simulink model "single_phase_csi"  (Simulink 6.1)
settings: Solver=ode23tb  StartTime=0.0  StopTime=0.03  MaxStep=1e-5  RelTol=1e-3  AbsTol=.01
libraries: powerlib x11
settings Model: LastModifiedBy=ThinkPad
settings DebuggingCC: SolverPrmCheckMsg=warning

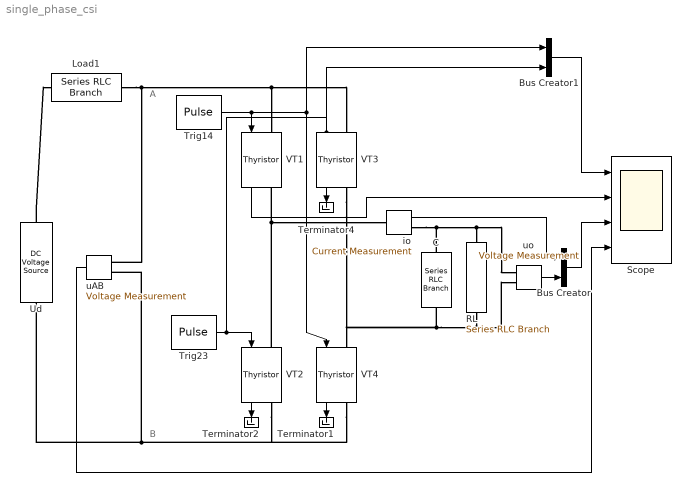
== system single_phase_csi ==
  note: A
  note: B
  Bus Creator : BusCreator  DialogController=Simulink.DDGSource_Bus  Inputs=2
  Bus Creator1 : BusCreator  DialogController=Simulink.DDGSource_Bus  Inputs=2
  C : powerlib/Elements/Series RLC Branch  Orientation=up  PhysicalDomain=powersysdomain  SubClassName=unknown  LeftPortType=p1  RightPortType=p1  LConnTagsString=__new0  RConnTagsString=__new0  Resistance=0  Inductance=0  Capacitance=800e-6  Measurements=None
  Load1 : powerlib/Elements/Series RLC Branch  Orientation=left  PhysicalDomain=powersysdomain  SubClassName=unknown  LeftPortType=p1  RightPortType=p1  LConnTagsString=__new0  RConnTagsString=__new0  Resistance=0  Inductance=0.002  Capacitance=inf  Measurements=None
  RL : powerlib/Elements/Series RLC Branch  Orientation=down  PhysicalDomain=powersysdomain  SubClassName=unknown  LeftPortType=p1  RightPortType=p1  LConnTagsString=__new0  RConnTagsString=__new0  Resistance=0.1  Inductance=50e-6  Capacitance=inf  Measurements=None
  Scope : Scope  NumInputPorts=4
      settings: TimeRange=0.005  YMin=-20~-400~-400~-200  YMax=20~400~400~200  SampleTime=1e-4
  Terminator1 : Terminator
      settings: Orientation=down
  Terminator2 : Terminator
      settings: Orientation=down
  Terminator4 : Terminator
      settings: Orientation=down
  Trig14 : DiscretePulseGenerator  PulseType=Time based  Amplitude=10  Period=0.001  PulseWidth=5
  Trig23 : DiscretePulseGenerator  PulseType=Time based  Amplitude=10  Period=0.001  PulseWidth=5  PhaseDelay=500e-6
  Ud : powerlib/Electrical Sources/DC Voltage Source  Orientation=up  Amplitude=50  Measurements=None
  VT{1..4} (4 alike) : powerlib/Power Electronics/Thyristor  Orientation=down  Ron=0.01  Lon=1e-6  Vf=0  IC=0  Rs=10  Cs=100e-9  Measurements=on
  io : powerlib/Measurements/Current Measurement  PhasorSimulation=off  OutputType=Complex  PSBequivalent=0
  uAB : powerlib/Measurements/Voltage Measurement  Orientation=left  PhasorSimulation=off  OutputType=Complex  PSBequivalent=0
  uo : powerlib/Measurements/Voltage Measurement  PhasorSimulation=off  OutputType=Complex  PSBequivalent=0
  wires:
  Trig14/1 -> VT1/1, VT4/1, Bus Creator1/1
  uo/1 -> Bus Creator/2
  Bus Creator/1 -> Scope/3
  io/1 -> Bus Creator/1
  Trig23/1 -> VT2/1, VT3/1, Bus Creator1/2
  Bus Creator1/1 -> Scope/1
  VT1/1 -> Scope/2
  uAB/1 -> Scope/4
  VT2/1 -> Terminator2/1
  VT4/1 -> Terminator1/1
  VT3/1 -> Terminator4/1
  connections:
  VT2/LConn1 -- VT1/RConn1 -- io/LConn1
  VT3/RConn1 -- VT4/LConn1 -- RL/RConn1 -- uo/LConn2 -- C/LConn1
  VT4/RConn1 -- VT2/RConn1 -- Ud/LConn1 -- uAB/LConn2
  Ud/RConn1 -- Load1/RConn1
  Load1/LConn1 -- VT3/LConn1 -- VT1/LConn1 -- uAB/LConn1
  io/RConn1 -- uo/LConn1 -- RL/LConn1 -- C/RConn1
